simulink model "base_model"  (R2013a)
settings: Solver=ode45  StartTime=0.0  StopTime=25  RelTol=1e-3
values from neighbouring files (symbols this model uses):
  A = [S3 S6 S7;S6 S8 S9; S7 S9 S10]    [LSQ_regression.m]
undefined symbols (not defined in the file or in its folder): C
settings Model: Creator=Aleksandr  LastModifiedBy=Aleksandr

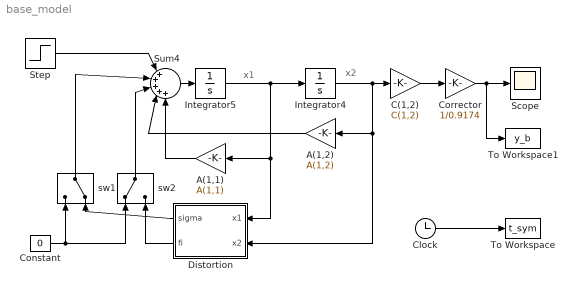
== system base_model ==
  note: x2
  note: x1
  A(1,1) : Gain  Gain=A(1,1)
  A(1,2) : Gain  Gain=A(1,2)
  C(1,2) : Gain  Gain=C(1,2)
  Clock : Clock
  Constant : Constant  Value=0
  Corrector : Gain  Gain=1/0.9174
  Distortion : Subsystem
  Integrator4 : Integrator
  Integrator5 : Integrator
  Scope : Scope
  Step : Step  SampleTime=0
  Sum4 : Sum  Inputs=|+++++
  To Workspace : ToWorkspace  VariableName=t_sym  SampleTime=-1
  To Workspace1 : ToWorkspace  VariableName=y_b  SampleTime=-1
  sw1 : ManualSwitch  CurrentSetting=0
  sw2 : ManualSwitch
  wires:
  C(1,2)/1 -> Corrector/1
  Sum4/1 -> Integrator5/1
  Integrator4/1 -> Distortion/2(x2), A(1,2)/1, C(1,2)/1
  Integrator5/1 -> Distortion/1(x1), A(1,1)/1, Integrator4/1
  A(1,1)/1 -> Sum4/5
  A(1,2)/1 -> Sum4/4
  Distortion/1(sigma) -> sw1/2
  Distortion/2(fi) -> sw2/2
  Constant/1 -> sw2/1, sw1/1
  sw2/1 -> Sum4/3
  sw1/1 -> Sum4/2
  Step/1 -> Sum4/1
  Corrector/1 -> To Workspace1/1, Scope/1
  Clock/1 -> To Workspace/1

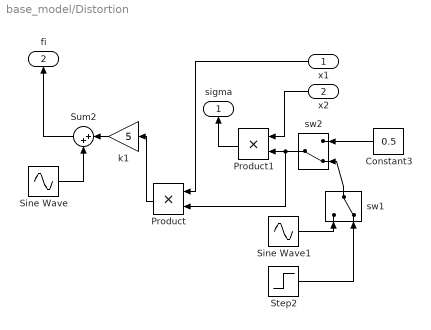
== system base_model/Distortion ==
  x1 : Inport
  x2 : Inport  Port=2
  Constant3 : Constant  Value=0.5
  Product : Product
  Product1 : Product
  Sine Wave : Sin  Frequency=pi/2  SampleTime=0
  Sine Wave1 : Sin  SampleTime=0
  Step2 : Step  Time=0  After=0.5  SampleTime=0
  Sum2 : Sum  Inputs=|++
  k1 : Gain  Gain=5
  sw1 : ManualSwitch  CurrentSetting=0
  sw2 : ManualSwitch  CurrentSetting=0
  sigma : Outport
  fi : Outport  Port=2
  wires:
  x1/1 -> Product/1
  Product1/1 -> sigma/1
  Sum2/1 -> fi/1
  Sine Wave1/1 -> sw1/1
  x2/1 -> Product1/1
  sw2/1 -> Product/2, Product1/2
  Step2/1 -> sw1/2
  Product/1 -> k1/1
  k1/1 -> Sum2/1
  Sine Wave/1 -> Sum2/2
  Constant3/1 -> sw2/1
  sw1/1 -> sw2/2
